simulink model "prova - Copia"  (R2022b)
settings: Solver=VariableStepAuto  StartTime=0.0  StopTime=.5  RelTol=1e-3
values from neighbouring files (symbols this model uses):
  da = 0    [Simulink_prova.m]
  dy = 0    [Simulink_prova.m]
  r = 1    [Simulink_prova.m]
libraries: cstblocks x2
settings Model: Creator=franc  LastModifiedBy=franc

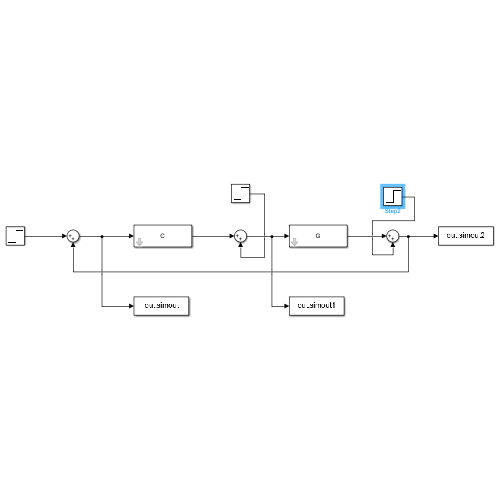
[thumbnail: Simulink's stored preview of the top-level diagram]
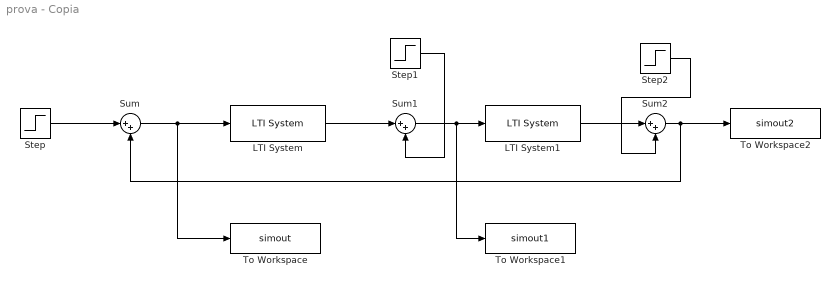
== system prova - Copia ==
  LTI System : cstblocks/LTI System  sys=C  IC=[]
  LTI System1 : cstblocks/LTI System  sys=G  IC=[]
  Step : Step  Time=0  After=r  SampleTime=0
  Step1 : Step  Time=0  After=da  SampleTime=0
  Step2 : Step  Time=0  After=dy  SampleTime=0
  Sum : Sum  Inputs=|++
  Sum1 : Sum  Inputs=|++
  Sum2 : Sum  Inputs=|++
  To Workspace : ToWorkspace  VariableName=simout  SaveFormat=Timeseries  SampleTime=-1
  To Workspace1 : ToWorkspace  VariableName=simout1  SaveFormat=Timeseries  SampleTime=-1
  To Workspace2 : ToWorkspace  VariableName=simout2  SaveFormat=Timeseries  SampleTime=-1
  wires:
  Step/1 -> Sum/1
  Sum/1 -> To Workspace/1, LTI System/1
  LTI System/1 -> Sum1/1
  Step1/1 -> Sum1/2
  Sum1/1 -> To Workspace1/1, LTI System1/1
  LTI System1/1 -> Sum2/1
  Step2/1 -> Sum2/2
  Sum2/1 -> To Workspace2/1, Sum/2
